simulink model "benchmark_1"  (R2016a)
settings: Solver=VariableStepAuto  StartTime=0.0  StopTime=time  RelTol=1e-3
values from neighbouring files (symbols this model uses):
  time_step = 0.01    [UAV_LAUNCHER_ASY_working_prot__v10.m]    (also in matlab_calc_actuator.m = 0.1; matlab_calc_tank_side.m = 7.0175)
libraries: fl_lib x9, nesl_utility x3
settings Model: Creator=Engr.Hammad  LastModifiedBy=Engr.Hammad

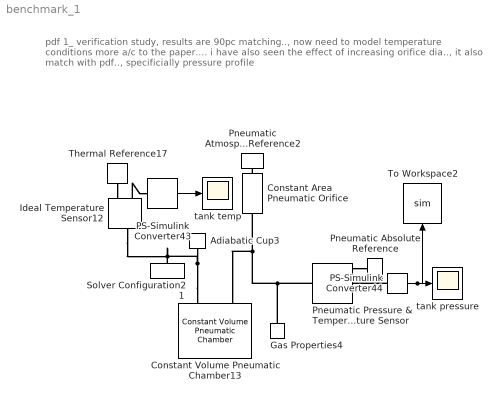
== system benchmark_1 ==
  note: pdf 1_ verification study, results are 90pc   matching.., now need to model temperature conditions more a/c to the paper....
      | i have also seen the effect of increasing orifice dia.., it also match with pdf.., specificially pressure profile
  Adiabatic Cup3 : fl_lib/Pneumatic/Pneumatic Elements/Adiabatic Cup
  Constant Area Pneumatic Orifice : fl_lib/Pneumatic/Pneumatic Elements/Constant Area Pneumatic Orifice  Cd=Cd  Area=At m^2  G_specify=off  G_priority=None  G=0 kg/s  Q1_specify=off  Q1_priority=None  Q1=0 J/s  Q2_specify=off  Q2_priority=None  Q2=0 J/s  p1_specify=off  p1_priority=None  p1=1e+5 Pa  p2_specify=off  p2_priority=None  p2=1e+5 Pa  T1_specify=off  T1_priority=None  T1=300 K  T2_specify=off  T2_priority=None  T2=300 K
  Constant Volume Pneumatic Chamber13 : fl_lib/Pneumatic/Pneumatic Elements/Constant Volume Pneumatic Chamber  Volume=V m^3  pressure_specify=on  pressure_priority=High  pressure=790 kPa  temperature_specify=on  temperature_priority=High  temperature=298.15 K  gas_flow_specify=off  gas_flow_priority=None  gas_flow=0 kg/s  heat_flow_specify=off  heat_flow_priority=None  heat_flow=0 J/s  heat_exch_flow_specify=off  heat_exch_flow_priority=None  heat_exch_flow=0 J/s
  Gas Properties4 : fl_lib/Pneumatic/Pneumatic Utilities/Gas Properties  c_p=1005 J/kg/K  c_v=717.95 J/kg/K  viscosity=18.21e-6 s*Pa  Pa=101325 Pa  Ta=293.15 K  range_error=2
  Ideal Temperature Sensor12 : fl_lib/Thermal/Thermal Sensors/Ideal Temperature Sensor
  PS-Simulink Converter43 : nesl_utility/PS-Simulink Converter  PhysicalDomain=network_engine_domain  SubClassName=ps_output  LeftPortType=input  RightPortType=output  PseudoPeriodic=off  Frequencies=[]  Unit=K  AffineConversion=on
  PS-Simulink Converter44 : nesl_utility/PS-Simulink Converter  PhysicalDomain=network_engine_domain  SubClassName=ps_output  LeftPortType=input  RightPortType=output  PseudoPeriodic=off  Frequencies=[]  Unit=1  AffineConversion=off
  Pneumatic Atmospheric Reference2 : fl_lib/Pneumatic/Pneumatic Elements/Pneumatic Atmospheric Reference
  Pneumatic Absolute Reference : fl_lib/Pneumatic/Pneumatic Elements/Pneumatic Absolute Reference
  Pneumatic Pressure & Temperature Sensor : fl_lib/Pneumatic/Pneumatic Sensors/Pneumatic Pressure & Temperature Sensor
  Solver Configuration21 : nesl_utility/Solver Configuration  PhysicalDomain=network_engine_domain  SubClassName=solver  LeftPortType=input  RightPortType=generic  Accelerate=off  Tones=[]  Harmonics=[]  SimulateNoise=off  Profile=off  UseLocalSampling=off  EnableSwitchedLinearOptims=on  FrequencyDomain=off  UseCCode=off  RelTol=0.001  AbsTol=1e-06  MinStep=1e-09  ToWorkspace=off  RevertToSquareIcSolve=off  NumHomotopyIterations=100  PhasorMode=off  PhasorModeNumHarmonics=1  OverrideAbsTol=off  DoDC=off  ResidualTolerance=1e-09  UseLocalSolver=off  LocalSolverChoice=NE_BACKWARD_EULER_ADVANCER  LocalSolverSampleTime=0.001  DoFixedCost=off  MaxNonlinIter=3  MaxModeIter=2  LinearAlgebra=Sparse  DelaysMemoryBudget=1024  AutomaticFiltering=on  FilteringTimeConstant=0.001
  Thermal Reference17 : fl_lib/Thermal/Thermal Elements/Thermal Reference
  To Workspace2 : ToWorkspace  VariableName=sim  SaveFormat=Structure With Time  SampleTime=time_step
  tank pressure : Scope
  "tank temp " : Scope
  wires:
  PS-Simulink Converter43/1 -> "tank temp "/1
  PS-Simulink Converter44/1 -> To Workspace2/1, tank pressure/1
  connections:
  Pneumatic Pressure & Temperature Sensor/LConn1 -- Constant Volume Pneumatic Chamber13/LConn1 -- Constant Area Pneumatic Orifice/LConn1 -- Gas Properties4/RConn1
  Constant Volume Pneumatic Chamber13/LConn2 -- Ideal Temperature Sensor12/LConn1 -- Solver Configuration21/RConn1 -- Adiabatic Cup3/LConn1
  Thermal Reference17/LConn1 -- Ideal Temperature Sensor12/RConn1
  Pneumatic Pressure & Temperature Sensor/RConn1 -- Pneumatic Absolute Reference/LConn1
  Constant Area Pneumatic Orifice/RConn1 -- Pneumatic Atmospheric Reference2/LConn1
  PS-Simulink Converter44/LConn1 -- Pneumatic Pressure & Temperature Sensor/RConn2
  Ideal Temperature Sensor12/RConn2 -- PS-Simulink Converter43/LConn1
